simulink library "tetherNnode_ul"  (R2018b)
settings: Solver=VariableStepAuto  StartTime=0.0  StopTime=10.0  RelTol=1e-3
values from neighbouring files (symbols this model uses):
  mass = 1000    [tetherNnode_ts.m]
undefined symbols (not defined in the file or in its folder): N
libraries: tetherBuoyAndWeight_ul x1, tetherDragForce_ul x1, tetherInternalForces_ul x1
settings Model: Creator=asiddiq2  LastModifiedBy=asiddiq2

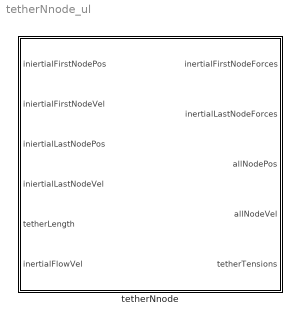
== system tetherNnode_ul ==
  tetherNnode : Subsystem  mask{gravAccl=10, rhoFluid=1, massBdy=mass, numNode=4, thrDia=0, thrRho=0, thrYoungs=0, thrZeta=0, thrCd=0}
      mask prompts: gravAccl "Gravitational acceleration"; rhoFluid "Fluid density"; massBdy "Vehicle Mass (kg)"; numNode "Number of nodes"; thrDia "Tether diameter"; thrRho "Tether density"; thrYoungs "Tether Youngs modulus"; thrZeta "Tether damping ratio"; thrCd "Tether drag coefficient"
      mask TypeOptions gravAccl: tetherNodalBuoyGravForces/gravAccl
      mask TypeOptions rhoFluid: tetherNodalDragForces/rhoFluid | tetherNodalBuoyGravForces/rhoFluid
      mask TypeOptions massBdy: tetherNodalinternalForces/massBdy
      mask TypeOptions numNode: tetherNodalBuoyGravForces/numNode | tetherNodalDragForces/numNode | tetherNodalinternalForces/numNode
      mask DialogControl ParameterGroupVar Prompt: Environment
      mask DialogControl Container4 Prompt: Vehicle
      mask DialogControl Container3 Prompt: Tether

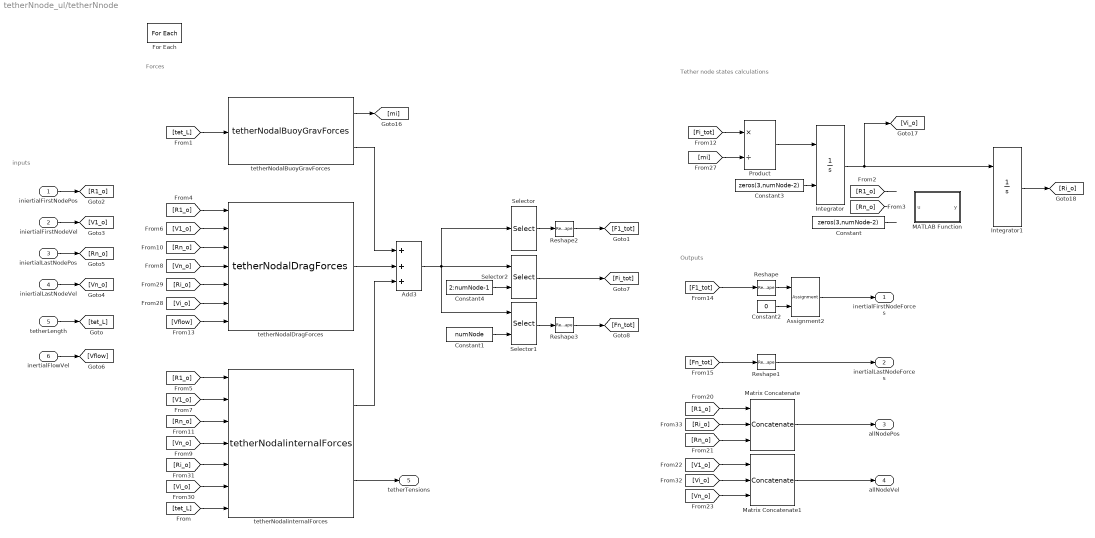
== system tetherNnode_ul/tetherNnode ==
  note: Outputs
  note: Forces
  note: inputs
  note: Tether node states calculations
  iniertialFirstNodePos : Inport  PortDimensions=[3,1]  Partition=on  PartitionDimension=2  PartitionWidth=1  PartitionOffset=0
  iniertialFirstNodeVel : Inport  Port=2  PortDimensions=[3,1]  Partition=on  PartitionDimension=2  PartitionWidth=1  PartitionOffset=0
  iniertialLastNodePos : Inport  Port=3  PortDimensions=[3,1]  Partition=on  PartitionDimension=2  PartitionWidth=1  PartitionOffset=0
  iniertialLastNodeVel : Inport  Port=4  PortDimensions=[3,1]  Partition=on  PartitionDimension=2  PartitionWidth=1  PartitionOffset=0
  tetherLength : Inport  Port=5  PortDimensions=[1,1]  Partition=on  PartitionDimension=2  PartitionWidth=1  PartitionOffset=0
  inertialFlowVel : Inport  Port=6
  Add3 : Sum  Inputs=+++
  Assignment2 : Assignment  NumberOfDimensions=2  DiagnosticForDimensions=Warning  IndexOptions=Index vector (dialog),Index vector (dialog)  Indices=3,1  OutputSizes=1,1
  Constant : Constant  Value=zeros(3,numNode-2)  VectorParams1D=off
  Constant1 : Constant  Value=numNode  VectorParams1D=off
  Constant2 : Constant  Value=0
  Constant3 : Constant  Value=zeros(3,numNode-2)  VectorParams1D=off
  Constant4 : Constant  Value=2:numNode-1  VectorParams1D=off
  For Each : ForEach  DisableCoverage=on  IterateSubsysMaskParameter=off,off,off,off,on,on,on,on,on  SubsysMaskParameterIterationDimension=1,1,1,1,2,2,2,2,2  IndexMode=One-based
  Integrator : Integrator  InitialConditionSource=external
  Integrator1 : Integrator  InitialConditionSource=external
  MATLAB Function : MATLAB Function  TreatAsAtomicUnit=on
  Matrix Concatenate : Concatenate  NumInputs=3  Mode=Multidimensional array  ConcatenateDimension=2
  Matrix Concatenate1 : Concatenate  NumInputs=3  Mode=Multidimensional array  ConcatenateDimension=2
  Product : Product  Inputs=*/
  Reshape{,1..3} (4 alike) : Reshape  OutputDimensionality=Column vector (2-D)
  Selector : Selector  NumberOfDimensions=2  InputPortWidth=3  IndexOptions=Select all,Index vector (dialog)  Indices=[1 3],1  OutputSizes=1,1
  Selector1 : Selector  NumberOfDimensions=2  InputPortWidth=3  IndexOptions=Select all,Index vector (port)  Indices=[1 3],N  OutputSizes=1,1
  Selector2 : Selector  NumberOfDimensions=2  InputPortWidth=3  IndexOptions=Select all,Index vector (port)  Indices=[1 3],[2:N-1]  OutputSizes=1,1
  tetherNodalBuoyGravForces : tetherBuoyAndWeight_ul/tetherNodalBuoyGravForces  rhoFluid=rhoFluid  gravAccl=gravAccl  numNode=numNode  diaTether=thrDia  rhoTether=thrRho
  tetherNodalDragForces : tetherDragForce_ul/tetherNodalDragForces  rhoFluid=rhoFluid  numNode=numNode  diaTether=thrDia  CdTether=thrCd
  tetherNodalinternalForces : tetherInternalForces_ul/tetherNodalinternalForces  massBdy=massBdy  numNode=numNode  diaTether=thrDia  youngsTether=thrYoungs  zetaTether=thrZeta
  inertialFirstNodeForces : Outport  PortDimensions=[3,1]  ConcatenationDimension=2
  inertialLastNodeForces : Outport  Port=2  PortDimensions=[3,1]  ConcatenationDimension=2
  allNodePos : Outport  Port=3  ConcatenationDimension=3
  allNodeVel : Outport  Port=4  ConcatenationDimension=3
  tetherTensions : Outport  Port=5  ConcatenationDimension=3
  wires:
  [Ri_o] -> tetherNodalDragForces/5
  tetherNodalinternalForces/2 -> tetherTensions/1
  [Fi_tot] -> Product/1
  [Rn_o] -> tetherNodalDragForces/3
  [Rn_o] -> ?
  Constant2/1 -> Assignment2/2
  Constant/1 -> ?
  [Rn_o] -> tetherNodalinternalForces/3
  [Vi_o] -> Matrix Concatenate1/2
  iniertialLastNodeVel/1 -> [Vn_o]
  [Vi_o] -> tetherNodalDragForces/6
  [Ri_o] -> tetherNodalinternalForces/5
  Reshape1/1 -> inertialLastNodeForces/1
  [Ri_o] -> Matrix Concatenate/2
  Product/1 -> Integrator/1
  [R1_o] -> ?
  Reshape/1 -> Assignment2/1
  [tet_L] -> tetherNodalinternalForces/7
  ? -> Integrator1/2
  Integrator1/1 -> [Ri_o]
  [R1_o] -> Matrix Concatenate/1
  [mi] -> Product/2
  Assignment2/1 -> inertialFirstNodeForces/1
  Matrix Concatenate1/1 -> allNodeVel/1
  [F1_tot] -> Reshape/1
  [V1_o] -> Matrix Concatenate1/1
  [Vflow] -> tetherNodalDragForces/7
  [R1_o] -> tetherNodalinternalForces/1
  Reshape2/1 -> [F1_tot]
  [Vi_o] -> tetherNodalinternalForces/6
  [Rn_o] -> Matrix Concatenate/3
  Reshape3/1 -> [Fn_tot]
  [tet_L] -> tetherNodalBuoyGravForces/1
  [Vn_o] -> tetherNodalDragForces/4
  [V1_o] -> tetherNodalDragForces/2
  inertialFlowVel/1 -> [Vflow]
  iniertialFirstNodePos/1 -> [R1_o]
  Selector2/1 -> [Fi_tot]
  [R1_o] -> tetherNodalDragForces/1
  [Vn_o] -> tetherNodalinternalForces/4
  [Fn_tot] -> Reshape1/1
  [V1_o] -> tetherNodalinternalForces/2
  Matrix Concatenate/1 -> allNodePos/1
  [Vn_o] -> Matrix Concatenate1/3
  iniertialFirstNodeVel/1 -> [V1_o]
  tetherLength/1 -> [tet_L]
  Integrator/1 -> [Vi_o], Integrator1/1
  iniertialLastNodePos/1 -> [Rn_o]
  Constant3/1 -> Integrator/2
  Add3/1 -> Selector2/1, Selector/1, Selector1/1
  Constant4/1 -> Selector2/2
  Constant1/1 -> Selector1/2
  Selector1/1 -> Reshape3/1
  Selector/1 -> Reshape2/1
  tetherNodalinternalForces/1 -> Add3/3
  tetherNodalDragForces/1 -> Add3/2
  tetherNodalBuoyGravForces/1 -> [mi]
  tetherNodalBuoyGravForces/2 -> Add3/1

== matlab function tetherNnode_ul/tetherNnode/MATLAB Function ==
  data: u input; y output
function y = fcn(u)

y = u;
